simulink model "sl"  (R2021a)
settings: Solver=VariableStepAuto  StartTime=0.0  StopTime=1  RelTol=1e-3
values from neighbouring files (symbols this model uses):
  Bl = 6.9    [OpenBoxLS.m]
  Cms = 594.85E-6    (= 0.00059485)    [OpenBoxLS.m]
  Le = 0.9E-3    (= 0.0009)    [OpenBoxLS.m]
  Mms = 13E-3    (= 0.013)    [OpenBoxLS.m]
  Re = 5.6    [OpenBoxLS.m]
  Rms = 0.6    [OpenBoxLS.m]
settings Model: Creator=padlewsk  LastModifiedBy=padlewsk

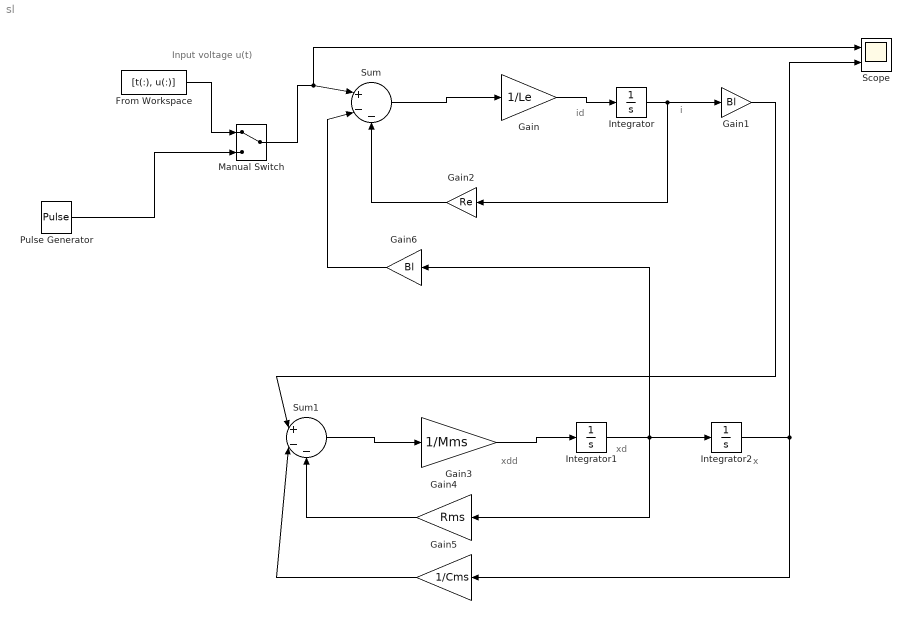
== system sl ==
  note: Input voltage u(t)
  note: i
  note: xdd
  note: xd
  note: x
  note: id
  From Workspace : FromWorkspace  VariableName=[t(:), u(:)]  SampleTime=0.001  OutputAfterFinalValue=Holding final value
  Gain : Gain  Gain=1/Le
  Gain1 : Gain  Gain=Bl
  Gain2 : Gain  Gain=Re
  Gain3 : Gain  Gain=1/Mms
  Gain4 : Gain  Gain=Rms
  Gain5 : Gain  Gain=1/Cms
  Gain6 : Gain  Gain=Bl
  Integrator : Integrator
  Integrator1 : Integrator
  Integrator2 : Integrator
  Manual Switch : ManualSwitch
  Pulse Generator : DiscretePulseGenerator  PulseType=Time based  Period=1  PulseWidth=5
  Scope : Scope  NumInputPorts=2
  Sum : Sum  Inputs=|+--
  Sum1 : Sum  Inputs=|+--
  wires:
  Sum/1 -> Gain/1
  Gain/1 -> Integrator/1
  Integrator/1 -> Gain2/1, Gain1/1
  Gain2/1 -> Sum/3
  Gain1/1 -> Sum1/1
  Sum1/1 -> Gain3/1
  Gain3/1 -> Integrator1/1
  Integrator1/1 -> Integrator2/1, Gain4/1, Gain6/1
  Integrator2/1 -> Gain5/1, Scope/2
  Gain6/1 -> Sum/2
  Gain5/1 -> Sum1/2
  Gain4/1 -> Sum1/3
  From Workspace/1 -> Manual Switch/1
  Manual Switch/1 -> Scope/1, Sum/1
  Pulse Generator/1 -> Manual Switch/2
